simulink model "SensingSubsystem"  (R2021b)
settings: Solver=VariableStepAuto  StartTime=0.0  StopTime=5 * chirp_params.cycle_period_us * 1e-6  RelTol=1e-3
undefined symbols (not defined in the file or in its folder): chirp_params, peak_detection_params, plot_params, waveform_params
libraries: hdlsllib x3, dspindex x3, dspsigops x2, simulink x1, dspxfrm3 x1, phasedwavlib x1, dspswit3 x1
settings Model: Creator=David  LastModifiedBy=David

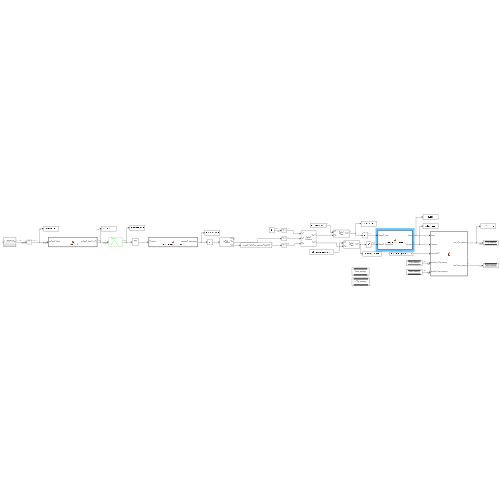
[thumbnail: Simulink's stored preview of the top-level diagram]
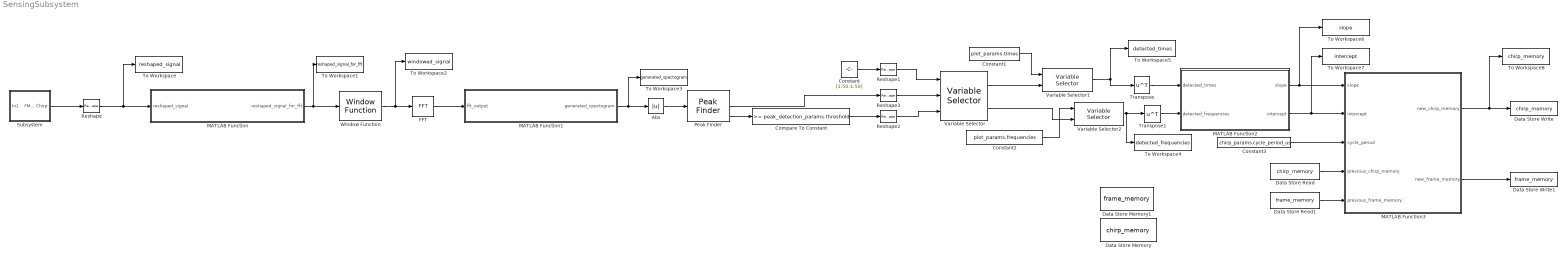
== system SensingSubsystem ==
  Abs : Abs
  Compare To Constant : simulink/Logic and Bit Operations/Compare To Constant  relop=>=  const=peak_detection_params.threshold  OutDataTypeStr=boolean
  Constant : Constant  Value=[1:50;1:50]  VectorParams1D=off
  Constant1 : Constant  Value=plot_params.times
  Constant2 : Constant  Value=plot_params.frequencies
  Constant3 : Constant  Value=chirp_params.cycle_period_us
  Data Store Memory : DataStoreMemory  DataStoreName=chirp_memory  ReadBeforeWriteMsg=warning  WriteAfterWriteMsg=warning  WriteAfterReadMsg=warning  InitialValue=zeros(2,6)  ShowAdditionalParam=off
  Data Store Memory1 : DataStoreMemory  DataStoreName=frame_memory  ReadBeforeWriteMsg=warning  WriteAfterWriteMsg=warning  WriteAfterReadMsg=warning  InitialValue=zeros(1,3)  VectorParams1D=off  ShowAdditionalParam=off
  Data Store Read : DataStoreRead  DataStoreName=chirp_memory  IndexOptions=Index vector (dialog)  Indices=1  OutputSizes=1
  Data Store Read1 : DataStoreRead  DataStoreName=frame_memory  IndexOptions=Index vector (dialog)  Indices=1  OutputSizes=1
  Data Store Write : DataStoreWrite  DataStoreName=chirp_memory  IndexOptions=Index vector (dialog)  Indices=1  OutputSizes=1
  Data Store Write1 : DataStoreWrite  DataStoreName=frame_memory  IndexOptions=Index vector (dialog)  Indices=1  OutputSizes=1
  FFT : dspxfrm3/FFT  FFTImplementation=Auto  CompMethod=Table lookup  TableOpt=NEW  TableOptActive=Speed  BitRevOrder=off  Normalize=off  InheritFFTLength=on  FFTLength=64  WrapInput=on  roundingMode=Floor  overflowMode=off  firstCoeffDataTypeStr=Inherit: Same word length as input  firstCoeffLastDataTypeStr=Inherit: Same word length as input  outputMin=[]  outputMax=[]
  MATLAB Function : MATLAB Function  TreatAsAtomicUnit=on
  MATLAB Function1 : MATLAB Function  TreatAsAtomicUnit=on
  MATLAB Function2 : MATLAB Function  TreatAsAtomicUnit=on
  MATLAB Function3 : MATLAB Function  TreatAsAtomicUnit=on
  Peak Finder : dspsigops/Peak Finder  polarity=Maxima  indexBase=One  outputIdx=on  outputVal=on  maxPeaks=2  NoiseDistinguish=off  thresh=1  roundingMode=Floor  overflowMode=off
      settings: SourceProductBaseCode=DS  allowOverrides=off
  Reshape : Reshape  OutputDimensionality=Customize  OutputDimensions=[50,50]
  Reshape1 : Reshape
  Reshape2 : Reshape
  Reshape3 : Reshape
  Subsystem : Subsystem
  To Workspace : ToWorkspace  VariableName=reshaped_signal  SampleTime=-1
      settings: MaxDataPoints=5
  To Workspace1 : ToWorkspace  VariableName=reshaped_signal_for_fft  SampleTime=-1
      settings: MaxDataPoints=5
  To Workspace2 : ToWorkspace  VariableName=windowed_signal  SampleTime=-1
      settings: MaxDataPoints=5
  To Workspace3 : ToWorkspace  VariableName=generated_spectogram  SampleTime=-1
      settings: MaxDataPoints=5
  To Workspace4 : ToWorkspace  VariableName=detected_frequencies  SampleTime=-1
      settings: MaxDataPoints=5
  To Workspace5 : ToWorkspace  VariableName=detected_times  SampleTime=-1
      settings: MaxDataPoints=5
  To Workspace6 : ToWorkspace  VariableName=slope  SampleTime=-1
      settings: MaxDataPoints=5
  To Workspace7 : ToWorkspace  VariableName=intercept  SampleTime=-1
      settings: MaxDataPoints=5
  To Workspace8 : ToWorkspace  VariableName=chirp_memory  SampleTime=-1
      settings: MaxDataPoints=5
  Transpose : Math  Operator=transpose  SaturateOnIntegerOverflow=on
  Transpose1 : Math  Operator=transpose  SaturateOnIntegerOverflow=on
  Variable Selector : dspindex/Variable Selector  NumInputs=2  rowsOrCols=Columns  IdxMode=Variable  Elements=[1 3]  ZerOneIdxMode=One-based  errmode=Clip Index  FillMode=on  FillValues=0
  Variable Selector1 : dspindex/Variable Selector  NumInputs=1  rowsOrCols=Rows  IdxMode=Variable  Elements=[1 3]  ZerOneIdxMode=One-based  errmode=Clip Index  FillMode=off  FillValues=0
  Variable Selector2 : dspindex/Variable Selector  NumInputs=1  rowsOrCols=Rows  IdxMode=Variable  Elements=[1 3]  ZerOneIdxMode=One-based  errmode=Clip Index  FillMode=off  FillValues=0
  Window Function : dspsigops/Window Function  winmode=Apply window to input  wintype=Hann  sampmode=Continuous  samptime=1  N=64  Rs=50  beta=10  winsamp=Symmetric  UserWindow=hamming  OptParams=off  UserParams={'symmetric'}  dataType=double  isSigned=on  wordLen=16  udDataType=sfix(16)  fracBitsMode=Best precision  numFracBits=15  roundingMode=Floor  overflowMode=off  numSidelobes=4  sidelobeLevel=-30
      settings: SourceProductBaseCode=DS
  wires:
  Reshape/1 -> MATLAB Function/1(reshaped_signal), To Workspace/1
  Subsystem/1(FMCW Chirp) -> Reshape/1
  MATLAB Function/1(reshaped_signal_for_fft) -> Window Function/1, To Workspace1/1
  Window Function/1 -> FFT/1, To Workspace2/1
  FFT/1 -> MATLAB Function1/1(fft_output)
  MATLAB Function1/1(generated_spectogram) -> Abs/1, To Workspace3/1
  Abs/1 -> Peak Finder/1
  Peak Finder/3 -> Compare To Constant/1
  Constant/1 -> Reshape1/1
  Compare To Constant/1 -> Reshape2/1
  Peak Finder/2 -> Reshape3/1
  Reshape1/1 -> Variable Selector/1
  Reshape3/1 -> Variable Selector/2
  Reshape2/1 -> Variable Selector/3
  Variable Selector/1 -> Variable Selector1/2
  Constant1/1 -> Variable Selector1/1
  Constant2/1 -> Variable Selector2/1
  Variable Selector/2 -> Variable Selector2/2
  Variable Selector2/1 -> To Workspace4/1, Transpose1/1
  Variable Selector1/1 -> Transpose/1, To Workspace5/1
  MATLAB Function2/1(slope) -> MATLAB Function3/1(slope), To Workspace6/1
  MATLAB Function2/2(intercept) -> MATLAB Function3/2(intercept), To Workspace7/1
  Constant3/1 -> MATLAB Function3/3(cycle_period)
  Data Store Read/1 -> MATLAB Function3/4(previous_chirp_memory)
  MATLAB Function3/1(new_chirp_memory) -> To Workspace8/1, Data Store Write/1
  Data Store Read1/1 -> MATLAB Function3/5(previous_frame_memory)
  MATLAB Function3/2(new_frame_memory) -> Data Store Write1/1
  Transpose/1 -> MATLAB Function2/1(detected_times)
  Transpose1/1 -> MATLAB Function2/2(detected_frequencies)

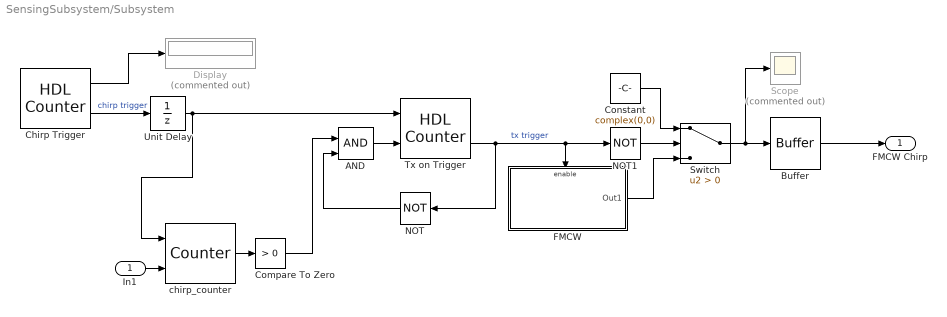
== system SensingSubsystem/Subsystem ==
  In1 : Inport
  AND : Logic  IconShape=distinctive  AllPortsSameDT=off  OutDataTypeStr=boolean
  Buffer : Buffer  N=int16(chirp_params.cycle_period_us * 1e-6 * waveform_params.sample_rate_Hz)  OutputFrames=off
  Chirp Trigger : hdlsllib/Sources/HDL Counter  CountType=Count limited  CountInit=1  CountStep=1  CountMax=waveform_params.sample_rate_Hz * waveform_params.sweep_time_s + chirp_params.num_samples_idle_time  CountFromType=Initial value  CountFrom=1  CountResetPort=on  CountLoadPort=off  CountEnbPort=off  CountDirPort=off  CountHitOutputPort=on  CountDataType=Unsigned  CountWordLen=16  CountFracLen=0  CountSampTime=1
  Compare To Zero : hdlsllib/Logic and Bit Operations/Compare To Zero  relop=>  OutDataTypeStr=boolean
      settings: SourceProductBaseCode=SL
  Constant : Constant  Value=complex(0,0)
  Display : Display  Commented=on
  FMCW : Subsystem
  NOT : Logic  Operator=NOT  IconShape=distinctive  AllPortsSameDT=off  OutDataTypeStr=boolean
  NOT1 : Logic  Operator=NOT  IconShape=distinctive  AllPortsSameDT=off  OutDataTypeStr=boolean
  Scope : Scope  Commented=on
  Switch : Switch  Criteria=u2 > Threshold
  Tx on Trigger : hdlsllib/Sources/HDL Counter  CountType=Count limited  CountInit=1  CountStep=1  CountMax=chirp_params.num_samples_idle_time  CountFromType=Initial value  CountFrom=1  CountResetPort=on  CountLoadPort=off  CountEnbPort=on  CountDirPort=off  CountHitOutputPort=on  CountDataType=Unsigned  CountWordLen=16  CountFracLen=0  CountSampTime=1
  Unit Delay : UnitDelay  SampleTime=-1  HasFrameUpgradeWarning=on
  chirp_counter : dspswit3/Counter  Direction=Up  CountEvent=Rising edge  CounterSize=User defined  MaxCount=frame_params.num_chirps  InitialCount=0  Output=Count  HitValue=32  ResetInput=on  SamplesPerFrame=1  Ts=1  CntDtype=int16  HitDtype=Logical
  FMCW Chirp : Outport
  wires:
  Buffer/1 -> FMCW Chirp/1
  chirp_counter/1 -> Compare To Zero/1
  In1/1 -> chirp_counter/2
  Chirp Trigger/2 -> Unit Delay/1  "chirp trigger"
  Tx on Trigger/2 -> NOT/1, FMCW/Enable, NOT1/1  "tx trigger"
  AND/1 -> Tx on Trigger/2
  Compare To Zero/1 -> AND/1
  NOT/1 -> AND/2
  Switch/1 -> Scope/1, Buffer/1
  FMCW/1(Out1) -> Switch/3
  NOT1/1 -> Switch/2
  Constant/1 -> Switch/1
  Chirp Trigger/1 -> Display/1
  Unit Delay/1 -> chirp_counter/1, Tx on Trigger/1

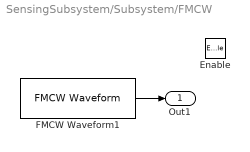
== system SensingSubsystem/Subsystem/FMCW ==
  Enable : EnablePort  StatesWhenEnabling=reset
  FMCW Waveform1 : phasedwavlib/FMCW Waveform  SampleRate=waveform_params.sample_rate_Hz  SweepTime=waveform_params.sweep_time_s  SweepBandwidth=waveform_params.sweep_BW_Hz  SweepDirection=Up  SweepInterval=Positive  OutputFormat=Samples  NumSamples=1  NumSweeps=waveform_params.num_sweeps  SimulateUsing=Interpreted execution
      settings: SourceProductBaseCode=AR
  Out1 : Outport
  wires:
  FMCW Waveform1/1 -> Out1/1

== matlab function SensingSubsystem/MATLAB Function1 ==
  data: fft_output input; generated_spectogram output; half_fft_size parameter
function generated_spectogram = remove_negative_frequencies(fft_output, half_fft_size)
   
generated_spectogram = fft_output(1:half_fft_size,:);

== matlab function SensingSubsystem/MATLAB Function ==
  data: reshaped_signal input; reshaped_signal_for_fft output; fft_size parameter
function reshaped_signal_for_fft = reshape_for_fft(reshaped_signal, fft_size)
   
reshaped_signal_for_fft = reshaped_signal(1:fft_size,:);

== matlab function SensingSubsystem/MATLAB Function2 ==
  data: detected_times input; slope output; detected_frequencies input; intercept output
function [slope,intercept] = compute_linear_model(detected_times,detected_frequencies)
    detected_times = detected_times(detected_times > 0);
    detected_frequencies = detected_frequencies(detected_frequencies > 0);
    if isempty(detected_frequencies)
        slope = 0;
        intercept = 0;
    else
        X = [ones(size(detected_times,2),1),detected_times.'];
        Y = detected_frequencies.';
        B = inv(X.' * X) * X.' * Y;
        slope = B(2);
        intercept = -1 * B(1)/B(2);
    end

== matlab function SensingSubsystem/MATLAB Function3 ==
  data: slope input; new_chirp_memory output; intercept input; cycle_period input; new_frame_memory output; previous_chirp_memory input; previous_frame_memory input
function [new_chirp_memory, new_frame_memory] = fcn(slope, intercept, cycle_period, previous_chirp_memory, previous_frame_memory)
    %protocol for chirp memory - [num chirp/slope samples, sum of slope samples, average slope, num chirp period samples, sum of chirp period samples, average chirp period;
    %                               previous chirp intercept, number of cycles since last detected chirp,0,0,0 ]
    %protocol for frame memory - [num samples, sum of samples, average]
    
    new_chirp_memory = zeros(2,6);
    new_frame_memory = zeros(1,3);
    
    %increment the number of cycles since last detected chirp
    new_chirp_memory(2,2) = previous_chirp_memory(2,2) + 1;

    if slope == 0
        new_chirp_memory = previous_chirp_memory;
        new_frame_memory = previous_frame_memory;
        new_chirp_memory(2,2) = previous_chirp_memory(2,2) + 1;
    elseif previous_chirp_memory(1,1) == 0
        %increment the chirp count
        new_chirp_memory(1,1) = 1;

        %compute the new average chirp slope
        new_chirp_memory(1,2) = slope;
        new_chirp_memory(1,3) = slope;


        %set the values for the previous chirp time and the number of
        %cycles since the last chirp
        new_chirp_memory(2,1) = intercept;
        new_chirp_memory(2,2) = 0;
    else
        %increment the chirp count and chirp period count
        new_chirp_memory(1,1) = previous_chirp_memory(1,1) + 1;
        new_chirp_memory(1,4) = previous_chirp_memory(1,4) + 1;

        %compute the new average chirp slope
        new_chirp_memory(1,2) = previous_chirp_memory(1,2) + slope;
        new_chirp_memory(1,3) = new_chirp_memory(1,2) / new_chirp_memory(1,1);

        %compute the new average chirp period
        new_chirp_cycle_time = intercept + new_chirp_memory(2,2) * cycle_period - previous_chirp_memory(2,1);
        new_chirp_memory(1,5) = previous_chirp_memory(1,5) + new_chirp_cycle_time;
        new_chirp_memory(1,6) = new_chirp_memory(1,5) / new_chirp_memory(1,4);

        %reset the values for the previous chirp time and the number of
        %cycles since the last chirp
        new_chirp_memory(2,1) = intercept;
        new_chirp_memory(2,2) = 0;
    end
